simulink model "VirtualDAQ_crashversion"  (R2021b)
settings: Solver=VariableStepAuto  StartTime=0.0  StopTime=inf  MaxStep=0.001  RelTol=1e-3
libraries: fl_lib x5, nesl_utility x3, simulink x2
(part 2 of 2)

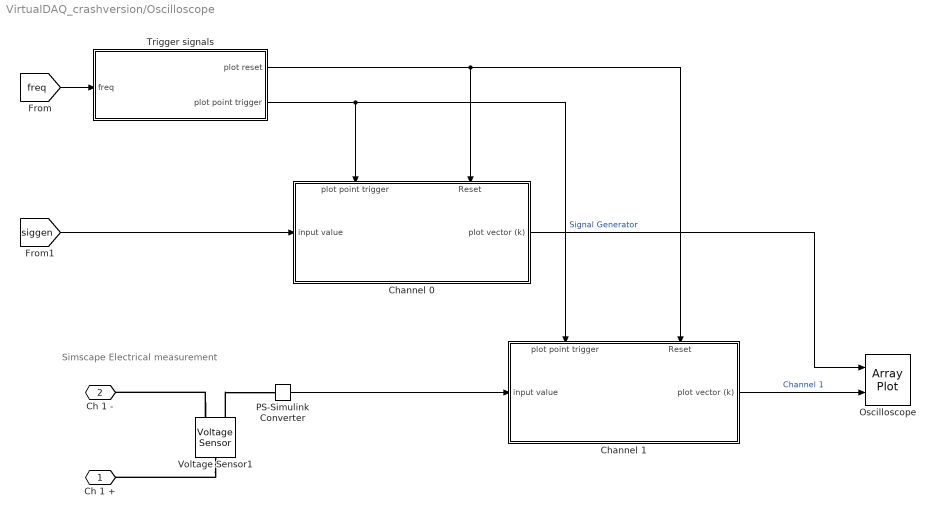
== system VirtualDAQ_crashversion/Oscilloscope ==
  note: Simscape Electrical measurement
  Channel 0 : Subsystem
      settings: PortSchema="{\"entries\":[{\"content\":{\"sides\":[{\"content\":{\"connectorIds\":[\"In1\"]},\"type\":\"ConnectorPlacement.EquallySpacedRectSide\",\"uuid\":\"56eea059-d5e9-4d95-b7d9-83a317b3103e\"},{\"content\":{\"connectorIds\":[\"Out1\"],\"side\":\"RIGHT\"},\"type\":\"ConnectorPlacement.EquallySpacedRectSide\",\"uuid\":\"fd8b8cd5-6def-4d8f-87ca-646372cc7fbe\"},{\"content\":{\"connectorIds\":[\"In2\",\"In3\"],\"side\":\"TOP\"},\"type\":\"ConnectorPlacement.EquallySpacedRectSide\",\"uuid\":\"3d9c38ee-b24b-466c-a7ac-a6d8a7456d51\"},{\"content\":{\"connectorIds\":[],\"side\":\"BOTTOM\"},\"type\":\"ConnectorPlacement.EquallySpacedRectSide\",\"uuid\":\"5165417f-5d3e-4abe-8dbf-33fc6b451c69\"}]},\"type\":\"ConnectorPlacement.EquallySpacedConnector\",\"uuid\":\"1d9824a8-6efd-49ff-b082-cf2ede19b4fd\"}],\"packageUris\":[\"http://schema.mathworks.com/mf0/Connector/R2020b\"],\"version\":\"1.0\"}"
  Channel 1 : Subsystem
      settings: PortSchema="{\"entries\":[{\"content\":{\"sides\":[{\"content\":{\"connectorIds\":[\"In1\"]},\"type\":\"ConnectorPlacement.EquallySpacedRectSide\",\"uuid\":\"56eea059-d5e9-4d95-b7d9-83a317b3103e\"},{\"content\":{\"connectorIds\":[\"Out1\"],\"side\":\"RIGHT\"},\"type\":\"ConnectorPlacement.EquallySpacedRectSide\",\"uuid\":\"fd8b8cd5-6def-4d8f-87ca-646372cc7fbe\"},{\"content\":{\"connectorIds\":[\"In2\",\"In3\"],\"side\":\"TOP\"},\"type\":\"ConnectorPlacement.EquallySpacedRectSide\",\"uuid\":\"3d9c38ee-b24b-466c-a7ac-a6d8a7456d51\"},{\"content\":{\"connectorIds\":[],\"side\":\"BOTTOM\"},\"type\":\"ConnectorPlacement.EquallySpacedRectSide\",\"uuid\":\"336136fa-2514-49ab-9e17-88caaca7366c\"}]},\"type\":\"ConnectorPlacement.EquallySpacedConnector\",\"uuid\":\"1d9824a8-6efd-49ff-b082-cf2ede19b4fd\"}],\"packageUris\":[\"http://schema.mathworks.com/mf0/Connector/R2020b\"],\"version\":\"1.0\"}"
  Oscilloscope : ArrayPlot  NumInputPorts=2  WindowPosition=[1282.000000,42.000000,1279.000000,1369.000000,]  PlotType=Line  AxesScaling=Manual  YLimits=[-5.1,5.1]  ShowLegend=on
  PS-Simulink Converter : nesl_utility/PS-Simulink Converter  PhysicalDomain=network_engine_domain  SubClassName=ps_output  LeftPortType=input  RightPortType=output  PseudoPeriodic=off  Frequencies=[]  Unit=inherit  AffineConversion=off
      settings: SourceProductBaseCode=PW,SS
  Trigger signals : Subsystem
  Voltage Sensor1 : fl_lib/Electrical/Electrical Sensors/Voltage Sensor
  Ch 1 + : PMIOPort  Side=Right
  Ch 1 - : PMIOPort  Port=2  Side=Right
  wires:
  PS-Simulink Converter/1 -> Channel 1/1(input value)
  Trigger signals/1("plot reset ") -> Channel 0/3(Reset), Channel 1/3(Reset)
  Channel 1/1(plot vector (k)) -> Oscilloscope/2  "Channel 1"
  Trigger signals/2(plot point trigger) -> Channel 0/2(plot point trigger), Channel 1/2(plot point trigger)
  [freq] -> Trigger signals/1(freq)
  Channel 0/1(plot vector (k)) -> Oscilloscope/1  "Signal Generator"
  [siggen] -> Channel 0/1(input value)
  connections:
  Voltage Sensor1/RConn2 -- Ch 1 -/RConn1
  Voltage Sensor1/RConn1 -- PS-Simulink Converter/LConn1
  Voltage Sensor1/LConn1 -- Ch 1 +/RConn1

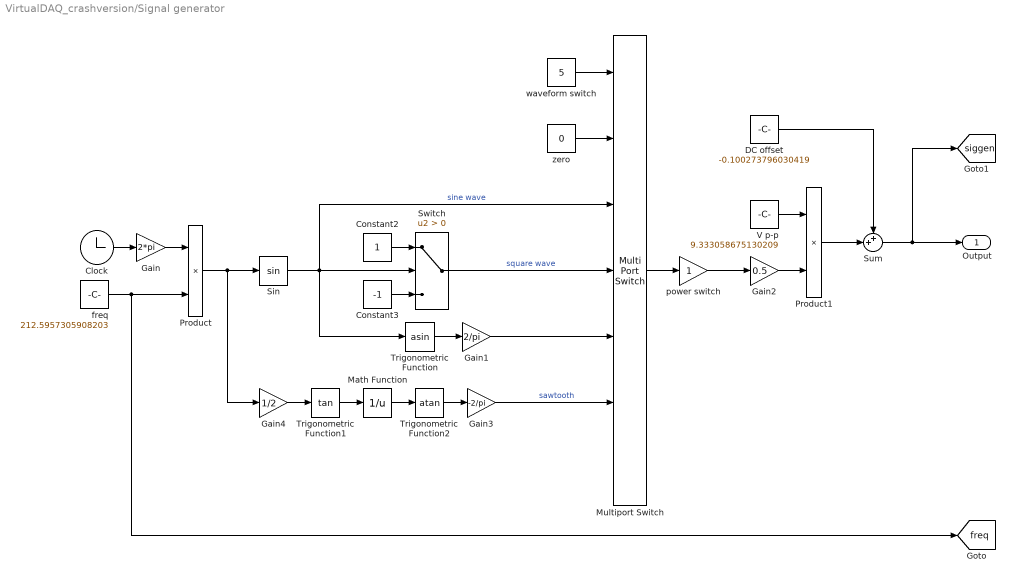
== system VirtualDAQ_crashversion/Signal generator ==
  Clock : Clock
  Constant2 : Constant  SampleTime=0
  Constant3 : Constant  Value=-1  SampleTime=0
  DC offset : Constant  Value=-0.100273796030419
  Gain : Gain  Gain=2*pi
  Gain1 : Gain  Gain=2/pi
  Gain2 : Gain  Gain=0.5
  Gain3 : Gain  Gain=-2/pi
  Gain4 : Gain  Gain=1/2
  Math Function : Math  Operator=reciprocal  SaturateOnIntegerOverflow=on
  Multiport Switch : MultiPortSwitch  DataPortOrder=Zero-based contiguous  Inputs=6  DiagnosticForDefault=None  zeroidx=on
  Product : Product
  Product1 : Product
  Sin : Trigonometry
  Sum : Sum  Inputs=++|
  Switch : Switch  Criteria=u2 > Threshold
  Trigonometric Function : Trigonometry  Operator=asin
  Trigonometric Function1 : Trigonometry  Operator=tan
  Trigonometric Function2 : Trigonometry  Operator=atan
  V p-p : Constant  Value=9.333058675130209  SampleTime=-1
  freq : Constant  Value=212.5957305908203  SampleTime=0
  power switch : Gain
  waveform switch : Constant  Value=5  SampleTime=0
  zero : Constant  Value=0  SampleTime=0
  Output : Outport
  tag scope: freq=global, siggen=global
  wires:
  Sin/1 -> Trigonometric Function/1, Multiport Switch/3, Switch/2  "sine wave"
  freq/1 -> [freq], Product/2
  Clock/1 -> Gain/1
  power switch/1 -> Gain2/1
  zero/1 -> Multiport Switch/2
  ? -> Multiport Switch/7
  Trigonometric Function/1 -> Gain1/1
  Constant2/1 -> Switch/1
  Constant3/1 -> Switch/3
  Gain2/1 -> Product1/2
  Product/1 -> Sin/1, Gain4/1
  Gain/1 -> Product/1
  Gain1/1 -> Multiport Switch/5
  waveform switch/1 -> Multiport Switch/1
  Math Function/1 -> Trigonometric Function2/1
  Trigonometric Function1/1 -> Math Function/1
  Trigonometric Function2/1 -> Gain3/1
  Gain4/1 -> Trigonometric Function1/1
  Multiport Switch/1 -> power switch/1
  Gain3/1 -> Multiport Switch/6  "sawtooth"
  V p-p/1 -> Product1/1
  Product1/1 -> Sum/2
  DC offset/1 -> Sum/1
  Switch/1 -> Multiport Switch/4  "square wave"
  Sum/1 -> [siggen], Output/1

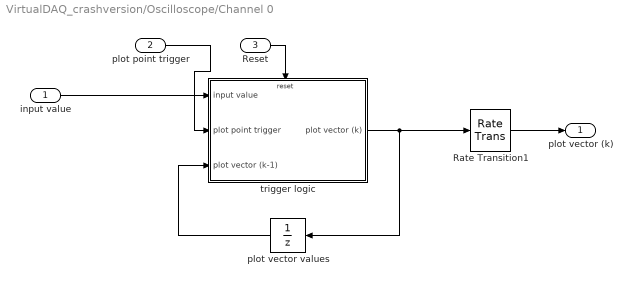
== system VirtualDAQ_crashversion/Oscilloscope/Channel 0 ==
  input value : Inport
  plot point trigger : Inport  Port=2
  Reset : Inport  Port=3
  Rate Transition1 : RateTransition  OutPortSampleTime=0.05
  plot vector values : UnitDelay  InitialCondition=zeros(250,1)  SampleTime=-1  HasFrameUpgradeWarning=on
  trigger logic : Subsystem  TreatAsAtomicUnit=on
  plot vector (k) : Outport
  wires:
  plot vector values/1 -> trigger logic/3(plot vector (k-1))
  plot point trigger/1 -> trigger logic/2(plot point trigger)
  Reset/1 -> trigger logic/Reset
  input value/1 -> trigger logic/1(input value)
  trigger logic/1(plot vector (k)) -> Rate Transition1/1, plot vector values/1
  Rate Transition1/1 -> plot vector (k)/1

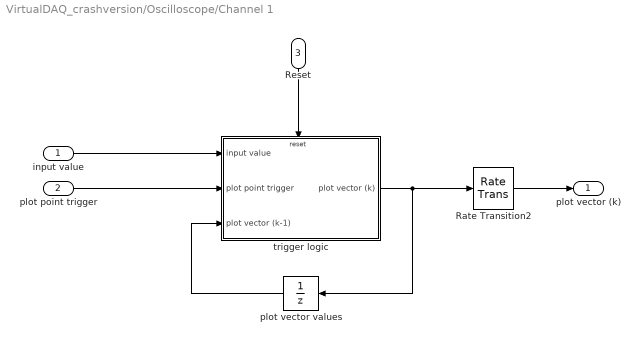
== system VirtualDAQ_crashversion/Oscilloscope/Channel 1 ==
  input value : Inport
  plot point trigger : Inport  Port=2
  Reset : Inport  Port=3
  Rate Transition2 : RateTransition  OutPortSampleTime=0.05
  plot vector values : UnitDelay  InitialCondition=zeros(250,1)  SampleTime=-1  HasFrameUpgradeWarning=on
  trigger logic : Subsystem  TreatAsAtomicUnit=on
  plot vector (k) : Outport
  wires:
  plot vector values/1 -> trigger logic/3(plot vector (k-1))
  plot point trigger/1 -> trigger logic/2(plot point trigger)
  trigger logic/1(plot vector (k)) -> Rate Transition2/1, plot vector values/1
  Reset/1 -> trigger logic/Reset
  input value/1 -> trigger logic/1(input value)
  Rate Transition2/1 -> plot vector (k)/1

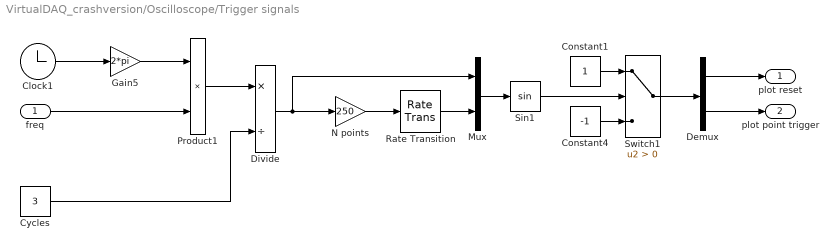
== system VirtualDAQ_crashversion/Oscilloscope/Trigger signals ==
  freq : Inport
  Clock1 : Clock
  Constant1 : Constant  SampleTime=0
  Constant4 : Constant  Value=-1  SampleTime=0
  Cycles : Constant  Value=3
  Demux : Demux  Outputs=2
  Divide : Product  Inputs=*/
  Gain5 : Gain  Gain=2*pi
  Mux : Mux  Inputs=2
  N points : Gain  Gain=250
  Product1 : Product
  Rate Transition : RateTransition  OutPortSampleTime=0.5e-5
  Sin1 : Trigonometry
  Switch1 : Switch  Criteria=u2 > Threshold
  "plot reset " : Outport
  plot point trigger : Outport  Port=2
  wires:
  Gain5/1 -> Product1/1
  Constant4/1 -> Switch1/3
  Clock1/1 -> Gain5/1
  Sin1/1 -> Switch1/2
  Constant1/1 -> Switch1/1
  freq/1 -> Product1/2
  Product1/1 -> Divide/1
  Cycles/1 -> Divide/2
  Divide/1 -> Mux/1, N points/1
  N points/1 -> Rate Transition/1
  Mux/1 -> Sin1/1
  Switch1/1 -> Demux/1
  Demux/2 -> plot point trigger/1
  Demux/1 -> "plot reset "/1
  Rate Transition/1 -> Mux/2

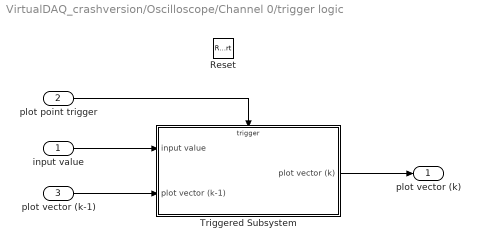
== system VirtualDAQ_crashversion/Oscilloscope/Channel 0/trigger logic ==
  input value : Inport
  plot point trigger : Inport  Port=2
  plot vector (k-1) : Inport  Port=3
  Reset : ResetPort  DisableCoverage=on
  Triggered Subsystem : Subsystem  TreatAsAtomicUnit=on
  plot vector (k) : Outport
  wires:
  plot point trigger/1 -> Triggered Subsystem/Trigger
  input value/1 -> Triggered Subsystem/1(input value)
  Triggered Subsystem/1(plot vector (k)) -> plot vector (k)/1
  plot vector (k-1)/1 -> Triggered Subsystem/2(plot vector (k-1))

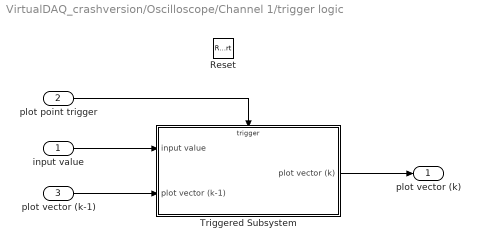
== system VirtualDAQ_crashversion/Oscilloscope/Channel 1/trigger logic ==
  input value : Inport
  plot point trigger : Inport  Port=2
  plot vector (k-1) : Inport  Port=3
  Reset : ResetPort  DisableCoverage=on
  Triggered Subsystem : Subsystem  TreatAsAtomicUnit=on
  plot vector (k) : Outport
  wires:
  plot point trigger/1 -> Triggered Subsystem/Trigger
  input value/1 -> Triggered Subsystem/1(input value)
  Triggered Subsystem/1(plot vector (k)) -> plot vector (k)/1
  plot vector (k-1)/1 -> Triggered Subsystem/2(plot vector (k-1))

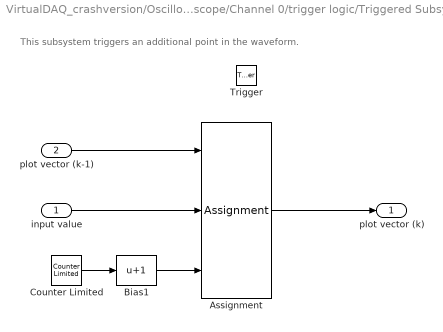
== system VirtualDAQ_crashversion/Oscilloscope/Channel 0/trigger logic/Triggered Subsystem ==
  note: This subsystem triggers an additional point in the waveform.
  input value : Inport
  plot vector (k-1) : Inport  Port=2
  Trigger : TriggerPort  VariantControl=(inherit)
  Assignment : Assignment  DiagnosticForDimensions=Warning  IndexOptions=Index vector (port)  Indices=1  OutputSizes=1
  Bias1 : Bias  Bias=1
  Counter Limited : simulink/Sources/Counter Limited  uplimit=250-1  tsamp=-1
  plot vector (k) : Outport
  wires:
  Assignment/1 -> plot vector (k)/1
  input value/1 -> Assignment/2
  Counter Limited/1 -> Bias1/1
  Bias1/1 -> Assignment/3
  plot vector (k-1)/1 -> Assignment/1

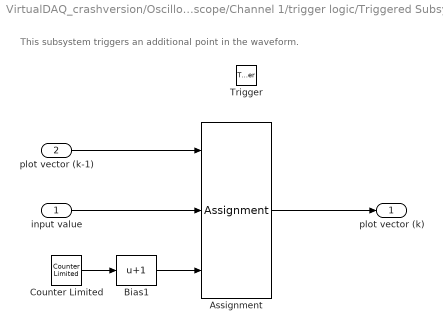
== system VirtualDAQ_crashversion/Oscilloscope/Channel 1/trigger logic/Triggered Subsystem ==
  note: This subsystem triggers an additional point in the waveform.
  input value : Inport
  plot vector (k-1) : Inport  Port=2
  Trigger : TriggerPort  VariantControl=(inherit)
  Assignment : Assignment  DiagnosticForDimensions=Warning  IndexOptions=Index vector (port)  Indices=1  OutputSizes=1
  Bias1 : Bias  Bias=1
  Counter Limited : simulink/Sources/Counter Limited  uplimit=250-1  tsamp=-1
  plot vector (k) : Outport
  wires:
  Assignment/1 -> plot vector (k)/1
  input value/1 -> Assignment/2
  Counter Limited/1 -> Bias1/1
  Bias1/1 -> Assignment/3
  plot vector (k-1)/1 -> Assignment/1
